simulink model "fullModelComplete"  (R2018a)
settings: Solver=ode45  StartTime=0.0  StopTime=10.0  RelTol=1e-3  EnableMultiTasking=on
PreLoadFcn:
  | load allParamValues.mat
values from neighbouring files (symbols this model uses):
  degConv = 57.2957795131    [allParamValues.mat]
  J = 0.000245    [allParamValues.mat]
  Ki = 2    [allParamValues.mat]
  Kp = 0.3    [allParamValues.mat]
  Ts = 0.01    [allParamValues.mat]
undefined symbols (not defined in the file or in its folder): sigbuilder_block
settings Model: Creator=jrivitus  LastModifiedBy=bneiswan
settings SolverCC: MaxConsecutiveZCs=25
settings DataIOCC: LimitDataPoints=on  SaveFormat=Array
settings OptimizationCC: ExpressionDepthLimit=2147483647  InitFltsAndDblsToZero=on  LifeSpan=inf
settings DebuggingCC: UnderspecifiedInitializationDetection=Classic  MergeDetectMultiDrivingBlocksExec=none  ParameterPrecisionLossMsg=none  FcnCallInpInsideContextMsg=warning  AllowSymbolicDim=off  StateNameClashWarn=warning  SFUnexpectedBacktrackingDiag=warning  SFNoUnconditionalDefaultTransitionDiag=warning  SFExecutionAtInitializationDiag=none
settings HardwareCC: ProdBitPerPointer=32  ProdBitPerSizeT=32  ProdBitPerPtrDiffT=32  ProdLargestAtomicFloat=None  ProdIntDivRoundTo=Undefined  ProdEndianess=Unspecified  ProdWordSize=32  ProdHWDeviceType=32-bit Generic
settings ModelReferenceCC: PropagateSignalLabelsOutOfModel=off
settings CodeAppCC: StateflowObjectComments=on
settings GRTTargetCC: TargetLangStandard=C89/C90 (ANSI)  GeneratePreprocessorConditionals=Disable all  CombineOutputUpdateFcns=off  GRTInterface=on
settings ConfigComp: CovMetricSettings=dw  CovHtmlReporting=on  CovSaveCumulativeToWorkspaceVar=on  CovSaveSingleToWorkspaceVar=on  CovExternalEMLEnable=off  CovSFcnEnable=off

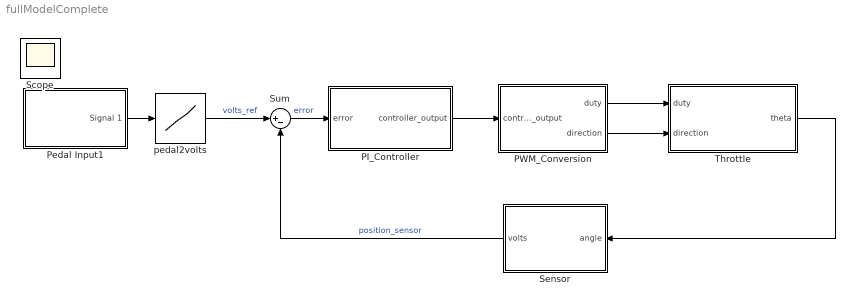
== system fullModelComplete ==
  PI_Controller : Subsystem
  PWM_Conversion : Subsystem
  Pedal Input1 : Subsystem  Tag=STV Subsys  LoadFcn=sigbuilder_block('load');  StartFcn=sigbuilder_block('start');  StopFcn=sigbuilder_block('stop');  ClipboardFcn=sigbuilder_block('clipboard');  mask(Sigbuilder block){tuvar=[0:10]}
      mask help: Sigbuilder GUI
      mask init:
      | if ~strcmp(get_param(bdroot(gcbh),'SimulationStatus'),'stopped') tuvar = sigbuilder_block('maskInit'); end
      settings: AttributesFormatString=0 - Pedal not pressed\n1 - Pedal fully pressed  CopyFcn=sigbuilder_block('copy');  DeleteFcn=sigbuilder_block('delete');  ModelCloseFcn=sigbuilder_block('modelClose');  PreSaveFcn=sigbuilder_block('preSave');  PauseFcn=sigbuilder_block('pause')  ContinueFcn=sigbuilder_block('continue')  NameChangeFcn=sigbuilder_block('namechange');  OpenFcn=sigbuilder_block('open',[437.6 199.2 550.4 400 ]);  CloseFcn=sigbuilder_block('close');
      mask Display: plot(0, 0, 100, 100,[2, 2, 32, 32, 2], [68, 8, 8, 68, 68],[32, 2], [38, 38], [32, 19, 2],[53, 60, 44], [32, 17, 17, 2],[16, 16, 31, 31]);txt = getActiveGroup(gcbh);text(2, 100, txt,'verticalAlignment', 'top');
  Sensor : Subsystem
  Sum : Sum  Inputs=|+-
  Throttle : Subsystem
  pedal2volts : Lookup_n-D  NumberOfTableDimensions=1  BreakpointsForDimension1=[0 1]  Table=[0.5 4.5]  RndMeth=Simplest  InputSameDT=on
  Scope : Scope
  wires:
  Pedal Input1/1(Signal 1) -> pedal2volts/1
  pedal2volts/1 -> Sum/1  "volts_ref"
  Sum/1 -> PI_Controller/1(error)  "error"
  PI_Controller/1(controller_output) -> PWM_Conversion/1(controller_output)
  PWM_Conversion/1("duty ") -> Throttle/1(duty)
  PWM_Conversion/2(" direction") -> Throttle/2(direction)
  Sensor/1(volts) -> Sum/2  "position_sensor"
  Throttle/1(theta) -> Sensor/1(angle)

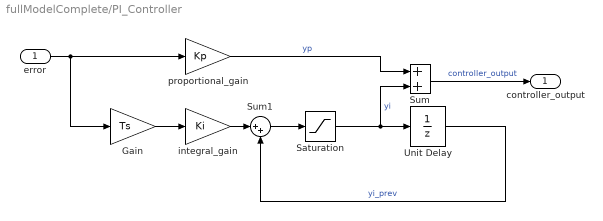
== system fullModelComplete/PI_Controller ==
  error : Inport  SampleTime=Ts
  Gain : Gain  Gain=Ts  SaturateOnIntegerOverflow=on  OutDataTypeStr=Inherit: Same as input  ParamDataTypeStr=Inherit: Same as input
  Saturation : Saturate  UpperLimit=1  LowerLimit=-1
      settings: AttributesFormatString=Max: %<UpperLimit>\nMin: %<LowerLimit>
  Sum : Sum  SaturateOnIntegerOverflow=on  InputSameDT=on  OutDataTypeStr=Inherit: Same as first input
  Sum1 : Sum  Inputs=|++  SaturateOnIntegerOverflow=on  InputSameDT=on  OutDataTypeStr=Inherit: Same as first input
  Unit Delay : UnitDelay  SampleTime=Ts
      settings: AttributesFormatString=yi0 = %<X0>\nSample time = %<SampleTime>
  integral_gain : Gain  Gain=Ki  SaturateOnIntegerOverflow=on  OutDataTypeStr=Inherit: Same as input  ParamDataTypeStr=Inherit: Same as input
  proportional_gain : Gain  Gain=Kp  SaturateOnIntegerOverflow=on  OutDataTypeStr=Inherit: Same as input  ParamDataTypeStr=Inherit: Same as input
  controller_output : Outport
  wires:
  Sum/1 -> controller_output/1  "controller_output"
  Saturation/1 -> Sum/2, Unit Delay/1  "yi"
  Sum1/1 -> Saturation/1
  Unit Delay/1 -> Sum1/2  "yi_prev"
  Gain/1 -> integral_gain/1
  integral_gain/1 -> Sum1/1
  proportional_gain/1 -> Sum/1  "yp"
  error/1 -> proportional_gain/1, Gain/1

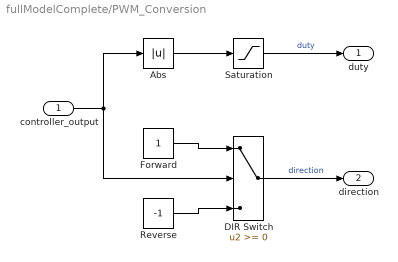
== system fullModelComplete/PWM_Conversion ==
  controller_output : Inport
  Abs : Abs
  DIR Switch : Switch
      settings: AttributesFormatString=Criteria: %<Criteria>\nThreshold: %<Threshold>
  Forward : Constant  OutDataTypeStr=double
  Reverse : Constant  Value=-1  OutDataTypeStr=double
  Saturation : Saturate  UpperLimit=1  LowerLimit=0
      settings: AttributesFormatString=%<LowerLimit> < duty < %<UpperLimit>
  "duty " : Outport
  " direction" : Outport  Port=2
  wires:
  controller_output/1 -> Abs/1, DIR Switch/2
  Forward/1 -> DIR Switch/1
  Reverse/1 -> DIR Switch/3
  DIR Switch/1 -> " direction"/1  "direction"
  Saturation/1 -> "duty "/1  "duty"
  Abs/1 -> Saturation/1

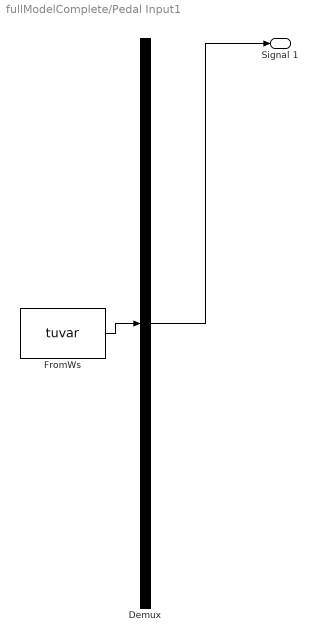
== system fullModelComplete/Pedal Input1 ==
  Demux : Demux  Tag=STV Demux  Outputs=1
  FromWs : FromWorkspace  Tag=STV FromWs  VariableName=tuvar  SampleTime=0
      SigBuilderData=|
      | common.afterFinalStr = 'Extrapolate'
      | common.sampleTime = 0
      | dataSet.timeRange = [0 10]
      | dataSet.name = 'Group 1'
      | sbobj.Groups.Name = 'Group 1'
      | sbobj.Groups.Signals.Name = 'Signal 1'
      | sbobj.Groups.Signals.XData = [0 2 2 6 6 10]
      | sbobj.Groups.Signals.YData = [0 0 0.8 0.8 0.2 0.2]
  Signal 1 : Outport  Tag=STV Outport
  wires:
  FromWs/1 -> Demux/1
  Demux/1 -> Signal 1/1

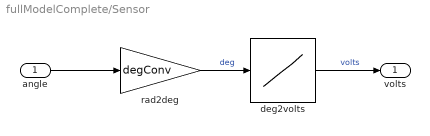
== system fullModelComplete/Sensor ==
  angle : Inport
  deg2volts : Lookup_n-D  NumberOfTableDimensions=1  BreakpointsForDimension1=[0 90]  Table=[0.5 4.5]  RndMeth=Simplest  InputSameDT=on
  rad2deg : Gain  Gain=degConv  SaturateOnIntegerOverflow=on  OutDataTypeStr=Inherit: Same as input  ParamDataTypeStr=Inherit: Same as input
  volts : Outport
  wires:
  rad2deg/1 -> deg2volts/1  "deg"
  deg2volts/1 -> volts/1  "volts"
  angle/1 -> rad2deg/1

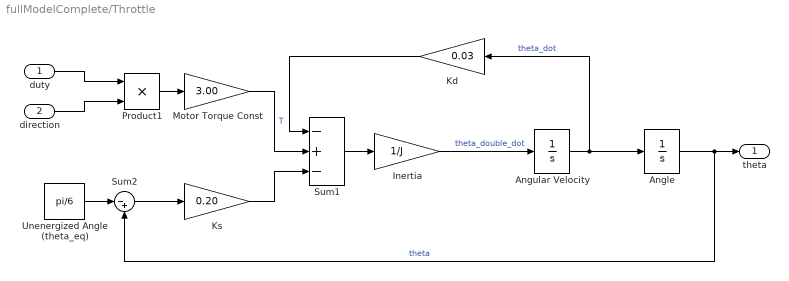
== system fullModelComplete/Throttle ==
  duty : Inport
  direction : Inport  Port=2
  Angle : Integrator  InitialCondition=pi/6  LimitOutput=on  UpperSaturationLimit=pi/2  LowerSaturationLimit=0
      settings: AttributesFormatString=Initial condition: %<InitialCondition>\n%<LowerSaturationLimit> <= theta <= %<UpperSaturationLimit>
  Angular Velocity : Integrator
      settings: AttributesFormatString=Initial condition: %<InitialCondition>
  Inertia : Gain  Gain=1/J  SaturateOnIntegerOverflow=on  OutDataTypeStr=Inherit: Same as input  ParamDataTypeStr=Inherit: Same as input
  Kd : Gain  Gain=0.03  SaturateOnIntegerOverflow=on  OutDataTypeStr=Inherit: Same as input  ParamDataTypeStr=Inherit: Same as input
  Ks : Gain  Gain=0.20  SaturateOnIntegerOverflow=on  OutDataTypeStr=Inherit: Same as input  ParamDataTypeStr=Inherit: Same as input
  Motor Torque Const : Gain  Gain=3.00  SaturateOnIntegerOverflow=on  OutDataTypeStr=Inherit: Same as input  ParamDataTypeStr=Inherit: Same as input
  Product1 : Product  SaturateOnIntegerOverflow=on  OutDataTypeStr=Inherit: Same as first input
  Sum1 : Sum  Inputs=-+-  SaturateOnIntegerOverflow=on
  Sum2 : Sum  Inputs=|-+  SaturateOnIntegerOverflow=on
  Unenergized Angle (theta_eq) : Constant  Value=pi/6
  theta : Outport
  wires:
  Ks/1 -> Sum1/3
  Kd/1 -> Sum1/1
  Motor Torque Const/1 -> Sum1/2  "T"
  duty/1 -> Product1/1
  direction/1 -> Product1/2
  Sum1/1 -> Inertia/1
  Inertia/1 -> Angular Velocity/1  "theta_double_dot"
  Angular Velocity/1 -> Kd/1, Angle/1  "theta_dot"
  Angle/1 -> Sum2/2, theta/1  "theta"
  Sum2/1 -> Ks/1
  Unenergized Angle (theta_eq)/1 -> Sum2/1
  Product1/1 -> Motor Torque Const/1
